simulink model "impedance_control"  (Simulink 9.0)
settings: Solver=FixedStepAuto  StartTime=0.0  StopTime=10.0  FixedStep=Ts  RelTol=1e-3
InitFcn:
  | setenv('YARP_ROBOT_NAME','iCubGazeboV2_5');
  | 
  | Ts = 0.01;
  | ROBOT_DOF = 23;
  | 
  | Kp = 1.5 * ones(ROBOT_DOF, 1);
  | Kd = 0.5 *  ones(ROBOT_DOF, 1);
  | 
  | refMask = zeros(ROBOT_DOF, 1);
  | %refMask(4) = 1; %l_shoulder_pitch
  | %refMask(7) = 1;
libraries: WBToolboxLibrary x8
settings Model: SuppressorTable=22 serialization::archive 11 0 6 0 0 0 11 0  Creator=dferigo  LastModifiedBy=dferigo
settings DataIOCC: SaveFormat=Dataset
settings OptimizationCC: LifeSpan=auto
settings DebuggingCC: UnderspecifiedInitializationDetection=Simplified  MergeDetectMultiDrivingBlocksExec=error  SFUnexpectedBacktrackingDiag=error  SFNoUnconditionalDefaultTransitionDiag=error  SFExecutionAtInitializationDiag=warning
settings HardwareCC: ProdBitPerPointer=64  ProdBitPerSizeT=64  ProdBitPerPtrDiffT=64  ProdLargestAtomicFloat=Float  ProdIntDivRoundTo=Zero  ProdEndianess=LittleEndian  ProdWordSize=64  ProdHWDeviceType=Intel->x86-64 (Windows64)
settings ModelReferenceCC: PropagateSignalLabelsOutOfModel=on
settings CodeAppCC: StateflowObjectComments=off
settings GRTTargetCC: TargetLangStandard=C99 (ISO)
settings ConfigComp: CovMetricSettings=dwe  CovHtmlReporting=off  CovSaveCumulativeToWorkspaceVar=off  CovSaveSingleToWorkspaceVar=off  CovExternalEMLEnable=on

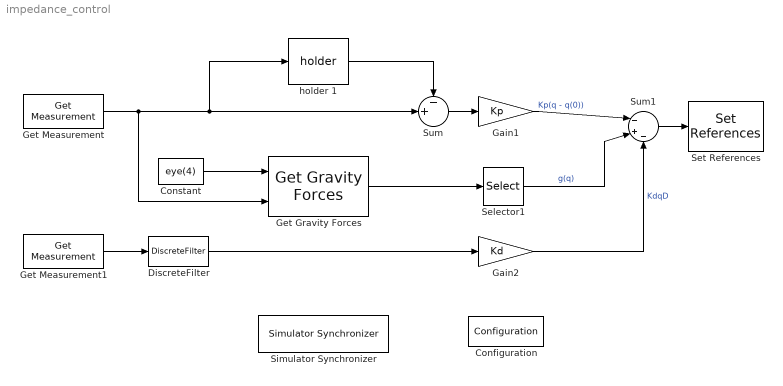
== system impedance_control ==
  Configuration : WBToolboxLibrary/Utilities/Configuration  ConfigSource=Mask  ConfigObject='WBTConfigRobot'  RobotName='icubSim'  UrdfFile='model.urdf'  ControlledJoints={'torso_pitch','torso_roll','torso_yaw','l_shoulder_pitch','l_shoulder_roll','l_shoulder_yaw','l_elbow','r_shoulder_pitch','r_shoulder_roll','r_shoulder_yaw','r_elbow','l_hip_pitch','l_hip_roll','l_hip_yaw','l_knee','l_ankle_pitch','l_ankle_roll','r_hip_pitch','r_hip_roll','r_hip_yaw','r_knee','r_ankle_pitch','r_ankle_roll'};  ControlBoardsNames={'torso','left_arm','right_arm','left_leg','right_leg'}  LocalName='WBT'  GravityVector=[0,0,-9.81]
      settings: SourceProductName=Whole Body Toolbox
  Constant : Constant  Value=eye(4)
  DiscreteFilter : WBToolboxLibrary/Utilities/DiscreteFilter  filterType=FirstOrderLowPassFilter  numCoeffs=[0]  denCoeffs=[0]  Fc=3  Ts=Ts  orderMedianFilter=0  initStatus=off  y0=[0]  u0=[0]
      settings: SourceProductName=Whole Body Toolbox
  Gain1 : Gain  Gain=Kp
  Gain2 : Gain  Gain=Kd
  Get Gravity Forces : WBToolboxLibrary/wholeBodyModel/Dynamics/Get Gravity Forces
      settings: SourceProductName=Whole Body Toolbox
  Get Measurement : WBToolboxLibrary/wholeBodyStates/Get Measurement  measuredType=Joints Position
      settings: SourceProductName=Whole Body Toolbox
  Get Measurement1 : WBToolboxLibrary/wholeBodyStates/Get Measurement  measuredType=Joints Velocity
      settings: SourceProductName=Whole Body Toolbox
  Selector1 : Selector  InputPortWidth=ROBOT_DOF+6  IndexOptions=Index vector (dialog)  Indices=[7:ROBOT_DOF+6]  OutputSizes=1
  Set References : WBToolboxLibrary/wholeBodyActuators/Set References  controlType=Torque  refSpeed=50
      settings: SourceProductName=Whole Body Toolbox
  Simulator Synchronizer : WBToolboxLibrary/Utilities/Simulator Synchronizer  period=0.01  serverPortName='/clock/rpc'  clientPortName='/WBT_synchronizer/rpc:o'
      settings: SourceProductName=Whole Body Toolbox
  Sum : Sum  Inputs=-+|
  Sum1 : Sum  Inputs=|-+-
  holder 1 : WBToolboxLibrary/Utilities/holder 
      settings: SourceProductName=Whole Body Toolbox
  wires:
  holder 1/1 -> Sum/1
  Selector1/1 -> Sum1/2  "g(q)"
  Gain2/1 -> Sum1/3  "KdqD"
  Sum1/1 -> Set References/1
  Gain1/1 -> Sum1/1  "Kp(q - q(0))"
  Constant/1 -> Get Gravity Forces/1
  Sum/1 -> Gain1/1
  Get Measurement1/1 -> DiscreteFilter/1
  DiscreteFilter/1 -> Gain2/1
  Get Gravity Forces/1 -> Selector1/1
  Get Measurement/1 -> holder 1/1, Sum/2, Get Gravity Forces/2
